simulink model "T1E5"  (R2013a)
settings: Solver=ode45  StartTime=0.0  StopTime=20  RelTol=1e-3
settings Model: Creator=Sudip Sinha  LastModifiedBy=Sudip Sinha

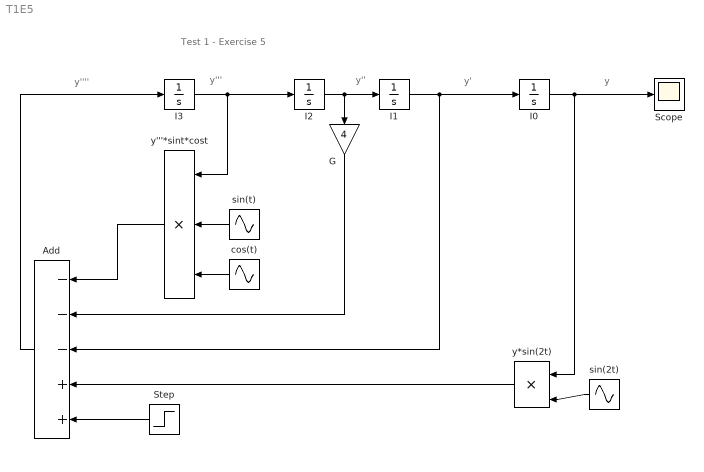
== system T1E5 ==
  note: Test 1 - Exercise 5
  note: y''''
  note: y
  note: y'''
  note: y''
  note: y'
  Add : Sum  Inputs=---++
  G : Gain  Gain=4
  I0 : Integrator  InitialCondition=3
  I1 : Integrator  InitialCondition=-2
  I2 : Integrator  InitialCondition=2
  I3 : Integrator  InitialCondition=-1
  Scope : Scope
      settings: ShowLegends=on
  Step : Step  After=0.1  SampleTime=0
  cos(t) : Sin  Phase=pi/2  SampleTime=0
  sin(2t) : Sin  Frequency=2  SampleTime=0
  sin(t) : Sin  SampleTime=0
  y'''*sint*cost : Product  Inputs=3
  y*sin(2t) : Product
  wires:
  I2/1 -> I1/1, G/1
  I0/1 -> y*sin(2t)/1, Scope/1
  I1/1 -> Add/3, I0/1
  G/1 -> Add/2
  Step/1 -> Add/5
  I3/1 -> y'''*sint*cost/1, I2/1
  y'''*sint*cost/1 -> Add/1
  cos(t)/1 -> y'''*sint*cost/3
  sin(t)/1 -> y'''*sint*cost/2
  sin(2t)/1 -> y*sin(2t)/2
  y*sin(2t)/1 -> Add/4
  Add/1 -> I3/1
